simulink model "emldemo_process_signal"  (R2015a)
settings: Solver=FixedStepDiscrete  StartTime=0.0  StopTime=1  RelTol=1e-3
libraries: simulink x1
settings Model: CovSFcnEnable=off  Creator=The MathWorks, Inc.  LastModifiedBy=ktrinh
settings OptimizationCC: ExpressionDepthLimit=2147483647
settings DebuggingCC: UnderspecifiedInitializationDetection=Classic  MergeDetectMultiDrivingBlocksExec=none  SolverPrmCheckMsg=warning  FcnCallInpInsideContextMsg=EnableAllAsWarning  StateNameClashWarn=warning  StrictBusMsg=Warning
settings SFSimCC: SimParseCustomCode=off
settings GRTTargetCC: CombineOutputUpdateFcns=off  GRTInterface=on

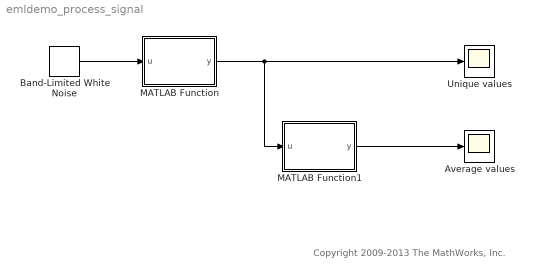
== system emldemo_process_signal ==
  note: Copyright 2009-2013 The MathWorks, Inc.
  Average values : Scope
      settings: TimeRange=auto  LimitDataPoints=on  MaxDataPoints=5000  SaveToWorkspace=off  YMin=-10  YMax=10  SampleTime=-1
  Band-Limited White Noise : simulink/Sources/Band-Limited White Noise  Cov=[0.1 0.2 0.3 0.4 0.5 0.6 0.1 0.2 0.3]  Ts=0.1  seed=[2223334]
  MATLAB Function : MATLAB Function  TreatAsAtomicUnit=on
      settings: PermitHierarchicalResolution=ParametersOnly
  MATLAB Function1 : MATLAB Function  TreatAsAtomicUnit=on
      settings: PermitHierarchicalResolution=ParametersOnly
  Unique values : Scope
      settings: TimeRange=auto  LimitDataPoints=on  MaxDataPoints=5000  SaveToWorkspace=off  SaveName=ScopeData  YMin=-10  YMax=10  SampleTime=-1
  wires:
  Band-Limited White Noise/1 -> MATLAB Function/1(u)
  MATLAB Function/1(y) -> Unique values/1, MATLAB Function1/1(u)
  MATLAB Function1/1(y) -> Average values/1

== matlab function emldemo_process_signal/MATLAB Function1 ==
  data: u input; y output size=[1 9]
function y = avg(u)
%#codegen

if numel(u) == 1
    y = u;
else
    k = numel(u)/2;
    if k ~= floor(k)
        u = u(2:numel(u));
    end
    y = emldemo_navg(u,2);
end

== matlab function emldemo_process_signal/MATLAB Function ==
  data: u input; y output size=[1 9]
function y = uniquify(u)
%#codegen

y = emldemo_uniquetol(u,0.2);
